simulink model "block_ss"  (R2018a)
settings: Solver=VariableStepAuto  StartTime=0.0  StopTime=10  RelTol=1e-3
values from neighbouring files (symbols this model uses):
  A_val = double(A)    [Drone_SysId_2step.m]    (also in Drone_System.m; Drone_System_control.m; Drone_System_full.m; Drone_System_identification.m)
  B_val = double(B)    [Drone_SysId_2step.m]    (also in Drone_System.m; Drone_System_control.m; Drone_System_full.m; Drone_System_identification.m)
  D_val = double(D)    [Drone_SysId_2step.m]    (also in Drone_System.m; Drone_System_control.m; Drone_System_full.m; Drone_System_identification.m)
settings Model: Creator=ros  LastModifiedBy=ros

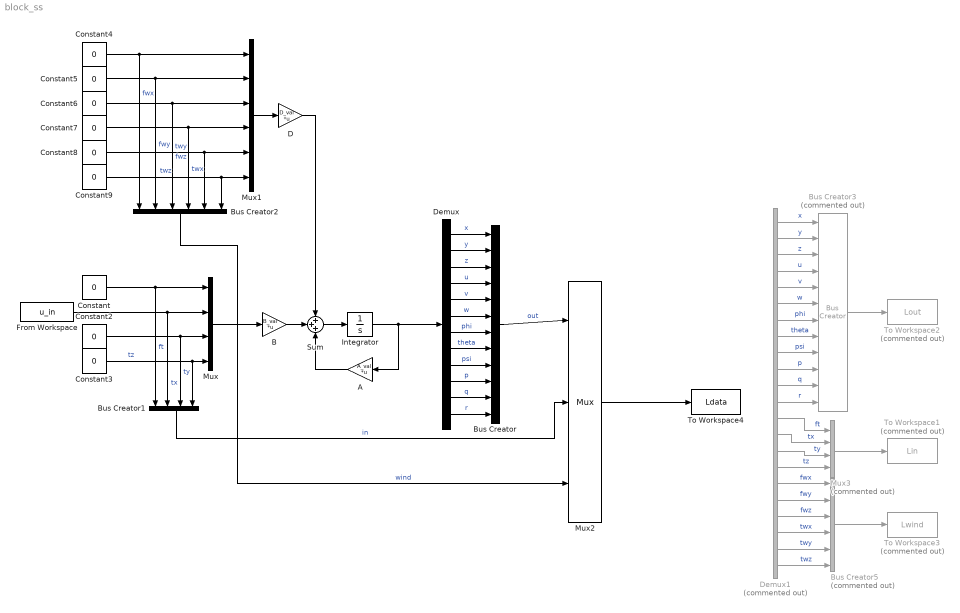
== system block_ss ==
  A : Gain  Gain=A_val  Multiplication=Matrix(K*u)
  B : Gain  Gain=B_val  Multiplication=Matrix(K*u)
  Bus Creator : BusCreator  Inputs=12
  Bus Creator1 : BusCreator  Inputs=4
  Bus Creator2 : BusCreator  Inputs=6
  Bus Creator3 : BusCreator  Commented=on  Inputs=12
  Bus Creator5 : BusCreator  Commented=on  Inputs=6
  Constant{,2..9} (9 alike) : Constant  Value=0
  D : Gain  Gain=D_val  Multiplication=Matrix(K*u)
  Demux : Demux  Outputs=12
  Demux1 : Demux  Commented=on  Outputs=22
  From Workspace : FromWorkspace  VariableName=u_in  SampleTime=0.001
  Integrator : Integrator  InitialCondition=[0 0 0 0 0 0 0 0 0 0 0 0]
  Mux : Mux
  Mux1 : Mux  Inputs=6
  Mux2 : Mux  Inputs=3
      settings: DisplayOption=signals
  Mux3 : Mux  Commented=on
  Sum : Sum  Inputs=+++
  To Workspace1 : ToWorkspace  Commented=on  VariableName=Lin  SaveFormat=Timeseries  SampleTime=-1
  To Workspace2 : ToWorkspace  Commented=on  VariableName=Lout  SaveFormat=Timeseries  SampleTime=-1
  To Workspace3 : ToWorkspace  Commented=on  VariableName=Lwind  SaveFormat=Timeseries  SampleTime=-1
  To Workspace4 : ToWorkspace  VariableName=Ldata  SaveFormat=Timeseries  SampleTime=-1
  wires:
  B/1 -> Sum/2
  A/1 -> Sum/3
  Sum/1 -> Integrator/1
  Integrator/1 -> A/1, Demux/1
  Constant/1 -> Mux/1, Bus Creator1/1  "ft"
  From Workspace/1 -> Mux/2, Bus Creator1/2  "tx"
  Constant2/1 -> Mux/3, Bus Creator1/3  "ty"
  Constant3/1 -> Mux/4, Bus Creator1/4  "tz"
  Mux/1 -> B/1
  Demux/1 -> Bus Creator/1  "x"
  Demux/2 -> Bus Creator/2  "y"
  Demux/3 -> Bus Creator/3  "z"
  Demux/4 -> Bus Creator/4  "u"
  Demux/5 -> Bus Creator/5  "v"
  Demux/6 -> Bus Creator/6  "w"
  Demux/7 -> Bus Creator/7  "phi"
  Demux/8 -> Bus Creator/8  "theta"
  Demux/9 -> Bus Creator/9  "psi"
  Demux/10 -> Bus Creator/10  "p"
  Demux/11 -> Bus Creator/11  "q"
  Demux/12 -> Bus Creator/12  "r"
  Bus Creator/1 -> Mux2/1  "out"
  Bus Creator1/1 -> Mux2/2  "in"
  Constant4/1 -> Bus Creator2/1, Mux1/1  "fwx"
  Constant5/1 -> Bus Creator2/2, Mux1/2  "fwy"
  Constant6/1 -> Bus Creator2/3, Mux1/3  "fwz"
  Constant7/1 -> Bus Creator2/4, Mux1/4  "twx"
  Constant8/1 -> Mux1/5, Bus Creator2/5  "twy"
  Constant9/1 -> Mux1/6, Bus Creator2/6  "twz"
  Mux1/1 -> D/1
  D/1 -> Sum/1
  Mux2/1 -> To Workspace4/1
  Bus Creator2/1 -> Mux2/3  "wind"
  Demux1/9 -> Bus Creator3/9  "psi"
  Demux1/2 -> Bus Creator3/2  "y"
  Demux1/10 -> Bus Creator3/10  "p"
  Demux1/8 -> Bus Creator3/8  "theta"
  Demux1/5 -> Bus Creator3/5  "v"
  Demux1/3 -> Bus Creator3/3  "z"
  Demux1/4 -> Bus Creator3/4  "u"
  Demux1/7 -> Bus Creator3/7  "phi"
  Demux1/12 -> Bus Creator3/12  "r"
  Demux1/6 -> Bus Creator3/6  "w"
  Demux1/1 -> Bus Creator3/1  "x"
  Demux1/11 -> Bus Creator3/11  "q"
  Bus Creator3/1 -> To Workspace2/1
  Mux3/1 -> To Workspace1/1
  Demux1/13 -> Mux3/1  "ft"
  Demux1/14 -> Mux3/2  "tx"
  Demux1/15 -> Mux3/3  "ty"
  Demux1/16 -> Mux3/4  "tz"
  Demux1/17 -> Bus Creator5/1  "fwx"
  Demux1/18 -> Bus Creator5/2  "fwy"
  Demux1/19 -> Bus Creator5/3  "fwz"
  Demux1/20 -> Bus Creator5/4  "twx"
  Demux1/21 -> Bus Creator5/5  "twy"
  Demux1/22 -> Bus Creator5/6  "twz"
  Bus Creator5/1 -> To Workspace3/1
